simulink model "SFcontroleur2"  (R2020a)
settings: Solver=VariableStepAuto  StartTime=0.0  StopTime=inf  RelTol=1e-3
settings Model: Creator=maxen  LastModifiedBy=maxen

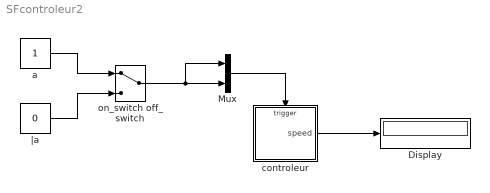
== system SFcontroleur2 ==
  Display : Display
  Mux : Mux  Inputs=2
  a : Constant
  controleur : Stateflow chart  TreatAsAtomicUnit=on
  on_switch off_switch : ManualSwitch
  |a : Constant  Value=0
  wires:
  |a/1 -> on_switch off_switch/2
  a/1 -> on_switch off_switch/1
  on_switch off_switch/1 -> Mux/2, Mux/1
  Mux/1 -> controleur/Trigger
  controleur/1(speed) -> Display/1

== stateflow chart SFcontroleur2/controleur ==
  settings: executeAtInitialization=1
  state On
    en:speed = 1;
  state Off
    en:speed = 0;
  On -> Off : off_switch
  (default) -> Off
  Off -> On : on_switch
  data: speed output
  events: on_switch input RISING_EDGE_EVENT; off_switch input FALLING_EDGE_EVENT
